simulink model "deploy_para_embarcar"  (R2023a)
settings: Solver=VariableStepAuto  StartTime=0.0  StopTime=10.0  RelTol=1e-3
model workspace (MAT data in the model file):
  bus_assignment_0 = 0
  centro_cordenadas_carro = 0
  curvatura_roda_para_coluna = 3.055
  forward_moviment = 1
undefined symbols (not defined in the file): aceleracao_lateral_max, constans_PID, desired_x, desired_y, max_velocity_longitudinal, pos_theta, pos_x, pos_y, vel_x
libraries: canmsglib x3, nvidiaCommlib x3, ros2lib x2, drivingvehiclecontroller x1, slpidlib x1
settings Model: DataDictionary=implementacao_deploy_23a.sldd  Creator=helenamandl  LastModifiedBy=lucas
settings DebuggingCC: UnderspecifiedInitializationDetection=Classic  MergeDetectMultiDrivingBlocksExec=none
settings ModelReferenceCC: PropagateSignalLabelsOutOfModel=off
settings RTWCC: GPUComputeCapability=5.0

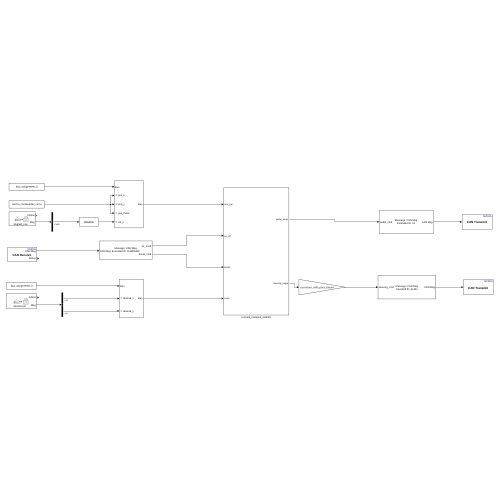
[thumbnail: Simulink's stored preview of the top-level diagram]
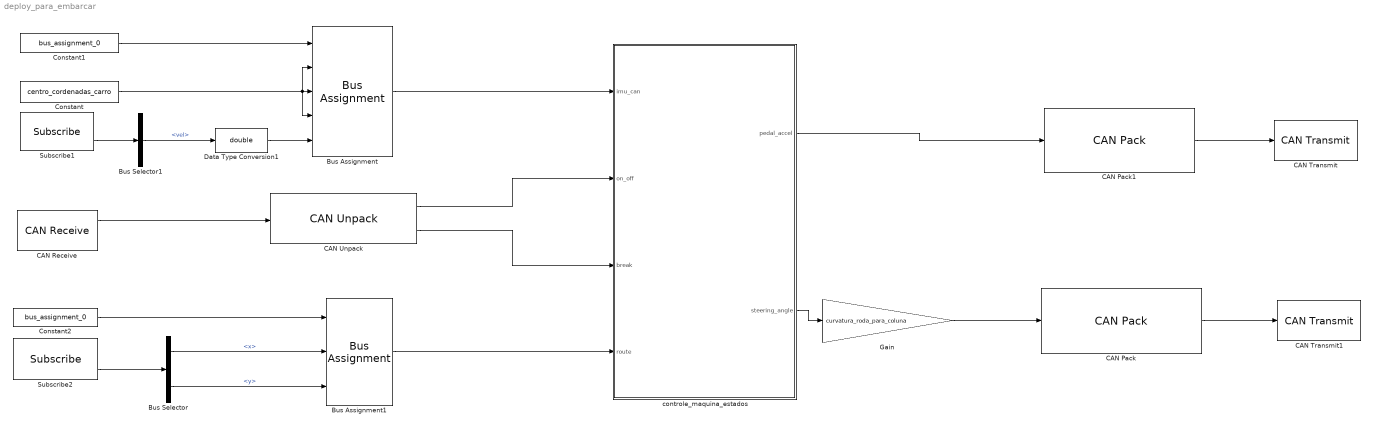
== system deploy_para_embarcar ==
  Bus Assignment : BusAssignment  AssignedSignals=pos_x,pos_y,pos_theta,vel_x
  Bus Assignment1 : BusAssignment  AssignedSignals=desired_x,desired_y
  Bus Selector : BusSelector  OutputSignals=pose.position.x,pose.position.y
  Bus Selector1 : BusSelector  OutputSignals=vel
  CAN Pack : canmsglib/CAN Pack  MsgList=(none)  MsgName=CAN Msg  MsgIDType=Standard (11-bit identifier)  MsgIdentifier=0x401  MsgLength=4  Remote=off  ApplyMinMax=off  BusOutput=on  SignalInfo={ 'steering_cmd', '24', '32', 'BE', 'signed', 'Standard', '0', '10000', '0', '-Inf', 'Inf' }
      settings: LibrarySourceBlock=c2000lib/Target Communication/CAN Pack  DataFormat=manually specified signals
  CAN Pack1 : canmsglib/CAN Pack  MsgList=(none)  MsgName=CAN Msg  MsgIDType=Extended (29-bit identifier)  MsgIdentifier=13  MsgLength=1  Remote=off  ApplyMinMax=off  BusOutput=on  SignalInfo={ 'pedal_cmd', '0', '8', 'LE', 'unsigned', 'Standard', '0', '1', '0', '0', '100' }
      settings: LibrarySourceBlock=c2000lib/Target Communication/CAN Pack  DataFormat=manually specified signals
  CAN Receive : nvidiaCommlib/CAN Receive  DeviceID=can0  SetupCAN=off  TypeofCAN=Real  OutputDataType=CAN Msg  IdentifierType=Extended (29-bit identifier)  MessageId=0x18ff1080  MsgLength=8  SampleTime=0.005  OutputError=off  OutputRemote=off  SimulateUsing=Code generation
      settings: SourceProductName=Communication
  CAN Transmit : nvidiaCommlib/CAN Transmit  DeviceID=vcan0  SetupCAN=off  TypeofCAN=Real  InputDataType=CAN Msg  BlockingMode_=off  BlockTimeout_=1  OutputStatus=off  IdentifierType=Standard (11-bit identifier)  MessageId=13  MsgLength=8  RemoteFrame=off  SimulateUsing=Code generation
      settings: SourceProductName=Communication
  CAN Transmit1 : nvidiaCommlib/CAN Transmit  DeviceID=vcan0  SetupCAN=off  TypeofCAN=Real  InputDataType=CAN Msg  BlockingMode_=off  BlockTimeout_=1  OutputStatus=off  IdentifierType=Extended (29-bit identifier)  MessageId=0x401  MsgLength=4  RemoteFrame=off  SimulateUsing=Code generation
      settings: SourceProductName=Communication
  CAN Unpack : canmsglib/CAN Unpack  MsgList=(none)  MsgName=CAN Msg  MsgIDType=Extended (29-bit identifier)  MsgIdentifier=0x18ff1080  MsgLength=4  SignalInfo={ 'hv_onoff', '0', '2', 'LE', 'signed', 'Standard', '0', '1', '0', '0', '3'; 'break_cmd', '3', '8', 'LE', 'signed', 'Standard', '1', '1', '0', '0', '255' }  IDPort=off  TimestampPort=off  ErrorPort=off  RemotePort=off  LengthPort=off  StatusPort=off  ApplyMinMax=off
      settings: LibrarySourceBlock=embeddedtargetslib/Host Communication/CAN Unpack
  Constant : Constant  Value=centro_cordenadas_carro
  Constant1 : Constant  Value=bus_assignment_0  OutDataTypeStr=Bus: bus_imu
  Constant2 : Constant  Value=bus_assignment_0  OutDataTypeStr=Bus: bus_route
  Data Type Conversion1 : DataTypeConversion  OutDataTypeStr=double  SaturateOnIntegerOverflow=off  RndMeth=Floor
  Gain : Gain  Gain=curvatura_roda_para_coluna
  Subscribe1 : ros2lib/Subscribe  topicSource=Specify your own  topic=/sbg/ekf_nav  messageType=geometry_msgs/TwistStamped  sampleTime=ts_ros2  QOSHistory=Keep last  QOSDepth=10  QOSReliability=Reliable  QOSDurability=Volatile  QOSDeadline=Inf  QOSLifespan=Inf  QOSLiveliness=Automatic  QOSLeaseDuration=Inf  QOSAvoidROSNamespaceConventions=off
  Subscribe2 : ros2lib/Subscribe  topicSource=Specify your own  topic=/teste/route  messageType=geometry_msgs/PoseStamped  sampleTime=ts_ros2  QOSHistory=Keep last  QOSDepth=10  QOSReliability=Reliable  QOSDurability=Volatile  QOSDeadline=Inf  QOSLifespan=Inf  QOSLiveliness=Automatic  QOSLeaseDuration=Inf  QOSAvoidROSNamespaceConventions=off
  controle_maquina_estados : Subsystem
  wires:
  CAN Pack/1 -> CAN Transmit1/1
  Gain/1 -> CAN Pack/1
  controle_maquina_estados/1(pedal_accel) -> CAN Pack1/1
  Bus Assignment1/1 -> controle_maquina_estados/4(route)
  CAN Unpack/1 -> controle_maquina_estados/2(on_off)
  Bus Assignment/1 -> controle_maquina_estados/1(imu_can)
  Bus Selector/2 -> Bus Assignment1/3  "<y>"
  Subscribe1/2 -> Bus Selector1/1
  Bus Selector1/1 -> Data Type Conversion1/1  "<vel>"
  CAN Pack1/1 -> CAN Transmit/1
  Constant2/1 -> Bus Assignment1/1
  CAN Unpack/2 -> controle_maquina_estados/3(break)
  Subscribe2/2 -> Bus Selector/1
  controle_maquina_estados/2(steering_angle) -> Gain/1
  Data Type Conversion1/1 -> Bus Assignment/5
  Bus Selector/1 -> Bus Assignment1/2  "<x>"
  Constant1/1 -> Bus Assignment/1
  CAN Receive/1 -> CAN Unpack/1
  Constant/1 -> Bus Assignment/2, Bus Assignment/4, Bus Assignment/3

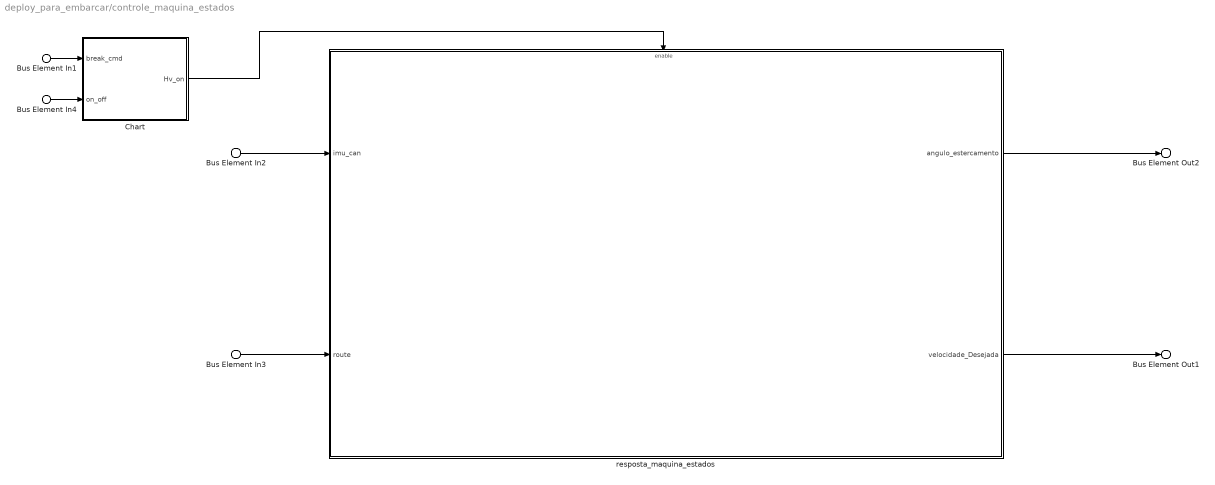
== system deploy_para_embarcar/controle_maquina_estados ==
  Bus Element In2 : Inport  PortName=imu_can
  Bus Element In4 : Inport  Port=2  PortName=on_off
  Bus Element In1 : Inport  Port=3  PortName=break
  Bus Element In3 : Inport  Port=4  PortName=route
  Chart : Stateflow chart  TreatAsAtomicUnit=on
  resposta_maquina_estados : Subsystem
  Bus Element Out1 : Outport  PortName=pedal_accel
  Bus Element Out2 : Outport  Port=2  PortName=steering_angle
  wires:
  Bus Element In1/1 -> Chart/1(break_cmd)
  resposta_maquina_estados/1(angulo_estercamento) -> Bus Element Out2/1
  resposta_maquina_estados/2(velocidade_Desejada) -> Bus Element Out1/1
  Chart/1(Hv_on) -> resposta_maquina_estados/Enable
  Bus Element In4/1 -> Chart/2(on_off)
  Bus Element In2/1 -> resposta_maquina_estados/1(imu_can)
  Bus Element In3/1 -> resposta_maquina_estados/2(route)

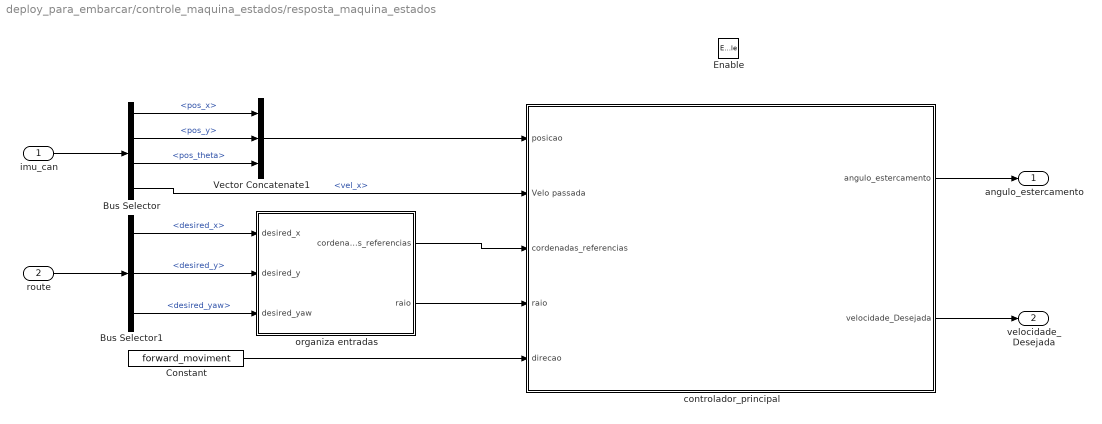
== system deploy_para_embarcar/controle_maquina_estados/resposta_maquina_estados ==
  imu_can : Inport
  route : Inport  Port=2
  Enable : EnablePort
  Bus Selector : BusSelector  OutputSignals=pos_x,pos_y,pos_theta,vel_x
  Bus Selector1 : BusSelector  OutputSignals=desired_x,desired_y,desired_yaw
  Constant : Constant  Value=forward_moviment
  Vector Concatenate1 : Concatenate  NumInputs=3
  controlador_principal : Subsystem
  organiza entradas : Subsystem
  angulo_estercamento : Outport
  velocidade_Desejada : Outport  Port=2
  wires:
  Bus Selector/4 -> controlador_principal/2(Velo passada)  "<vel_x>"
  controlador_principal/1(angulo_estercamento) -> angulo_estercamento/1
  Bus Selector/1 -> Vector Concatenate1/1  "<pos_x>"
  Bus Selector1/1 -> organiza entradas/1(desired_x)  "<desired_x>"
  Bus Selector/2 -> Vector Concatenate1/2  "<pos_y>"
  imu_can/1 -> Bus Selector/1
  Bus Selector1/2 -> organiza entradas/2(desired_y)  "<desired_y>"
  organiza entradas/1(cordenadas_referencias) -> controlador_principal/3(cordenadas_referencias)
  Bus Selector1/3 -> organiza entradas/3(desired_yaw)  "<desired_yaw>"
  route/1 -> Bus Selector1/1
  Bus Selector/3 -> Vector Concatenate1/3  "<pos_theta>"
  controlador_principal/2(velocidade_Desejada) -> velocidade_Desejada/1
  Vector Concatenate1/1 -> controlador_principal/1(posicao)
  Constant/1 -> controlador_principal/5(direcao)
  organiza entradas/2(raio) -> controlador_principal/4(raio)

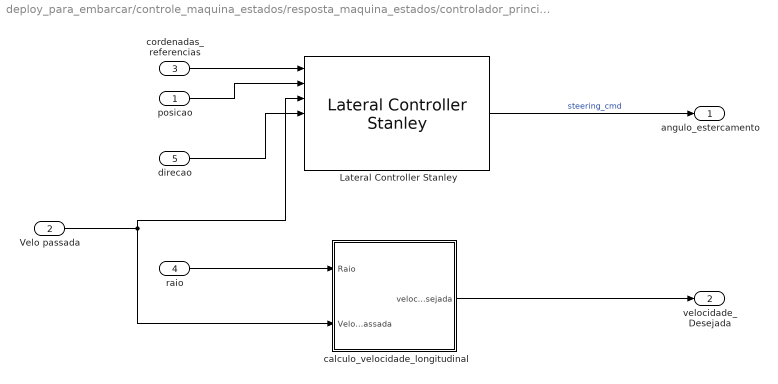
== system deploy_para_embarcar/controle_maquina_estados/resposta_maquina_estados/controlador_principal ==
  posicao : Inport
  Velo passada : Inport  Port=2
  cordenadas_referencias : Inport  Port=3
  raio : Inport  Port=4
  direcao : Inport  Port=5
  Lateral Controller Stanley : drivingvehiclecontroller/Lateral Controller Stanley  ModelType=Dynamic bicycle model  PositionGainF=stanley_kpfw  PositionGainR=stanley_kprv  YawRateGain=1  DelayGain=0.2  VehicleMass=230  Lf=1.4  Lr=1.6  TireStiffness=12e3  Wheelbase=wheelbase  MaxSteeringAngle=max_steering_angle
  calculo_velocidade_longitudinal : Subsystem
  angulo_estercamento : Outport  OutMax=[0]  PortDimensions=1
  velocidade_Desejada : Outport  Port=2
  wires:
  direcao/1 -> Lateral Controller Stanley/4
  posicao/1 -> Lateral Controller Stanley/2
  cordenadas_referencias/1 -> Lateral Controller Stanley/1
  calculo_velocidade_longitudinal/1(velocidade_desejada) -> velocidade_Desejada/1
  Velo passada/1 -> Lateral Controller Stanley/3, calculo_velocidade_longitudinal/2(Velo passada)
  raio/1 -> calculo_velocidade_longitudinal/1(Raio)
  Lateral Controller Stanley/1 -> angulo_estercamento/1  "steering_cmd"

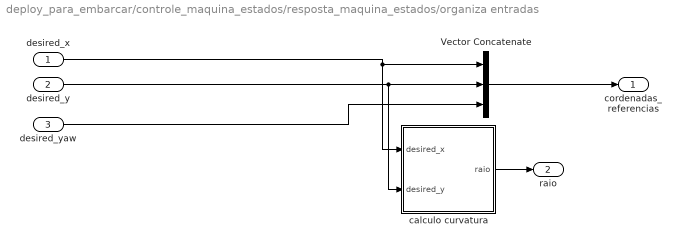
== system deploy_para_embarcar/controle_maquina_estados/resposta_maquina_estados/organiza entradas ==
  desired_x : Inport
  desired_y : Inport  Port=2
  desired_yaw : Inport  Port=3
  Vector Concatenate : Concatenate  NumInputs=3
  calculo curvatura : Subsystem
  cordenadas_referencias : Outport
  raio : Outport  Port=2
  wires:
  desired_yaw/1 -> Vector Concatenate/3
  Vector Concatenate/1 -> cordenadas_referencias/1
  desired_y/1 -> calculo curvatura/2(desired_y), Vector Concatenate/2
  desired_x/1 -> calculo curvatura/1(desired_x), Vector Concatenate/1
  calculo curvatura/1(raio) -> raio/1

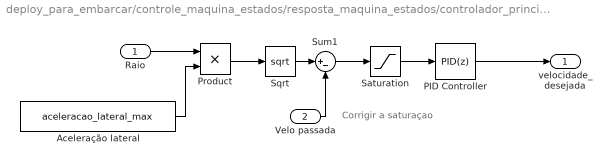
== system deploy_para_embarcar/controle_maquina_estados/resposta_maquina_estados/controlador_principal/calculo_velocidade_longitudinal ==
  note: Corrigir a saturaçao
  Raio : Inport
  Velo passada : Inport  Port=2
  Aceleração lateral : Constant  Value=aceleracao_lateral_max
  PID Controller : slpidlib/PID Controller  Controller=PID  Form=Parallel  TimeDomain=Discrete-time  UseExternalTs=off  SampleTime=-1  IntegratorMethod=Forward Euler  FilterMethod=Forward Euler  ControllerParametersSource=internal  P=constans_PID(1)  I=constans_PID(2)  UseKiTs=off  D=constans_PID(3)  N=constans_PID(4)  UseFilter=on  TunerSelectOption=Transfer Function Based (PID Tuner App)  InitialConditionSource=internal  InitialConditionForIntegrator=0  InitialConditionForFilter=0  DifferentiatorICPrevScaledInput=0  ExternalReset=none  TrackingMode=off  Kt=1  LimitOutput=off  SatLimitsSource=internal  UpperSaturationLimit=12  LowerSaturationLimit=-12  LinearizeAsGain=on  AntiWindupMode=none  Kb=1  LimitIntegrator=off  UpperIntegratorSaturationLimit=inf  LowerIntegratorSaturationLimit=-inf  POutMin=[]  POutMax=[]  IOutMin=[]  IOutMax=[]  DOutMin=[]  DOutMax=[]  NOutMin=[]  NOutMax=[]  SumOutMin=[]  SumOutMax=[]  SaturationOutMin=[]  SaturationOutMax=[]  PParamMin=[]  PParamMax=[]  IParamMin=[]  IParamMax=[]  DParamMin=[]  DParamMax=[]  NParamMin=[]  NParamMax=[]  KbParamMin=[]  KbParamMax=[]  KtParamMin=[]  KtParamMax=[]  KbOutMin=[]  KbOutMax=[]  KtOutMin=[]  KtOutMax=[]  IntegratorOutMin=[]  IntegratorOutMax=[]  FilterOutMin=[]  FilterOutMax=[]  SumI1OutMin=[]  SumI1OutMax=[]  SumI2OutMin=[]  SumI2OutMax=[]  SumI3OutMin=[]  SumI3OutMax=[]  SumI4OutMin=[]  SumI4OutMax=[]  SumDOutMin=[]  SumDOutMax=[]  DifferentiatorOutMin=[]  DifferentiatorOutMax=[]  FilterDiffOutCoefMin=[]  FilterDiffOutCoefMax=[]  ReciprocalOutMin=[]  ReciprocalOutMax=[]  SumDenOutMin=[]  SumDenOutMax=[]  SumNumOutMin=[]  SumNumOutMax=[]  DivideOutMin=[]  DivideOutMax=[]  UdiffTsProdOutMin=[]  UdiffTsProdOutMax=[]  NTsProdOutMin=[]  NTsProdOutMax=[]  UintegralTsProdOutMin=[]  UintegralTsProdOutMax=[]  UngainTsProdOutMin=[]  UngainTsProdOutMax=[]  ClampingZeroOutDataTypeStr=Inherit: Inherit via back propagation  ClampingZeroOutMin=[]  ClampingZeroOutMax=[]  FilterDenConstantOutDataTypeStr=Inherit: Inherit via back propagation  FilterDenConstantOutMin=[]  FilterDenConstantOutMax=[]  PCopyOutDataTypeStr=Inherit: Inherit via back propagation  PCopyOutMin=[]  PCopyOutMax=[]  NCopyOutDataTypeStr=Inherit: Inherit via back propagation  NCopyOutMin=[]  NCopyOutMax=[]  IntegratorContinuousStateAttributes=''  IntegratorStateMustResolveToSignalObject=off  IntegratorRTWStateStorageClass=Auto  FilterContinuousStateAttributes=''  FilterStateMustResolveToSignalObject=off  FilterRTWStateStorageClass=Auto  ParallelPVariant=InternalParameters  IdealPVariant=Disabled  IVariant=InternalParameters  DVariant=InternalParameters  IntegratorVariant=Discrete  SatVariant=Disabled  AWVariant=Passthrough  PCopyVariant=Disabled  TRVariant=Disabled  FdbkBlocksVariant=Forward  IdealPFdbkVariant=Disabled  SatFdbkVariant=Disabled  DerivativeFilterVariant=ForwardEulerFilter  NVariant=InternalParameters  NCopyVariant=Disabled  FilterICVariant=InternalICsFilter  IntegratorICVariant=InternalICs  ExternalResetVariant=Disabled  TRSumVariant=Passthrough  SumFdbkVariant=Disabled  SumVariant=Sum_PID  TsampFilterVariant=InternalTs  TsampNgainVariant=Passthrough  TsampIntegralVariant=Disabled_SignalSpec  ExternalSaturationOutDataTypeStr=Inherit: Same as second input
  Product : Product
  Saturation : Saturate  UpperLimit=max_velocity_longitudinal  LowerLimit=0
      settings: AttributesFormatString=Velocidade maxima do carro=%<UpperLimit>
  Sqrt : Sqrt
  Sum1 : Sum  Inputs=|+-
  velocidade_desejada : Outport
  wires:
  Saturation/1 -> PID Controller/1
  Sum1/1 -> Saturation/1
  PID Controller/1 -> velocidade_desejada/1
  Product/1 -> Sqrt/1
  Aceleração lateral/1 -> Product/2
  Sqrt/1 -> Sum1/1
  Raio/1 -> Product/1
  Velo passada/1 -> Sum1/2

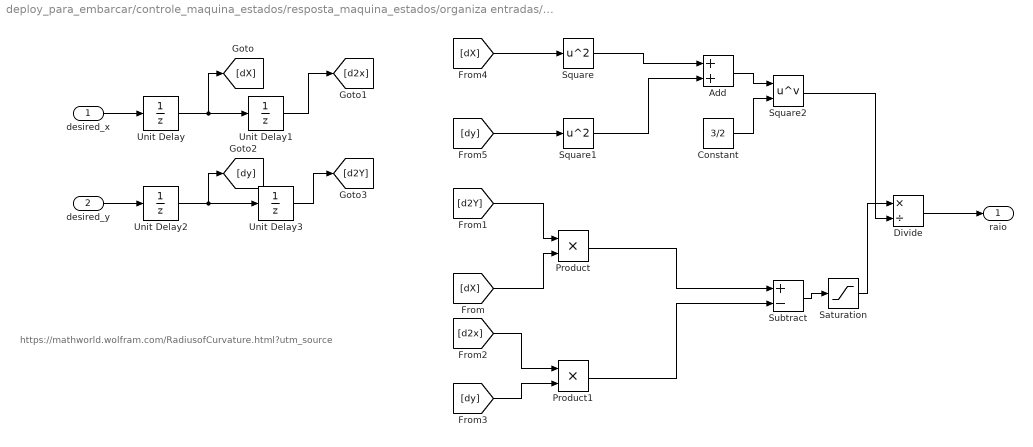
== system deploy_para_embarcar/controle_maquina_estados/resposta_maquina_estados/organiza entradas/calculo curvatura ==
  note: https://mathworld.wolfram.com/RadiusofCurvature.html?utm_source
  desired_x : Inport
  desired_y : Inport  Port=2
  Add : Sum
  Constant : Constant  Value=3/2
  Divide : Product  Inputs=*/
  Product : Product
  Product1 : Product
  Saturation : Saturate  UpperLimit=10000  LowerLimit=0.00001
  Square : Math  Operator=square
  Square1 : Math  Operator=square
  Square2 : Math  Operator=pow
  Subtract : Sum  Inputs=+-
  Unit Delay{,1..3} (4 alike) : UnitDelay  SampleTime=-1  HasFrameUpgradeWarning=on
  raio : Outport
  wires:
  [dX] -> Square/1
  [d2x] -> Product1/1
  desired_x/1 -> Unit Delay/1
  [dy] -> Product1/2
  Product/1 -> Subtract/1
  Unit Delay1/1 -> [d2x]
  Add/1 -> Square2/1
  Unit Delay/1 -> [dX], Unit Delay1/1
  Square1/1 -> Add/2
  [d2Y] -> Product/1
  [dy] -> Square1/1
  Product1/1 -> Subtract/2
  [dX] -> Product/2
  desired_y/1 -> Unit Delay2/1
  Unit Delay2/1 -> [dy], Unit Delay3/1
  Constant/1 -> Square2/2
  Unit Delay3/1 -> [d2Y]
  Divide/1 -> raio/1
  Square2/1 -> Divide/2
  Subtract/1 -> Saturation/1
  Saturation/1 -> Divide/1
  Square/1 -> Add/1

== stateflow chart deploy_para_embarcar/controle_maquina_estados/Chart ==
  state Idle
  state HV
    entry:
    Hv_on = 1;
  (default) -> Idle
  Idle -> HV : [on_off==true]
  HV -> Idle : [(on_off == false) || (break_cmd == true) ]
  data: break_cmd input; on_off input; Hv_on output
